simulink model "sliding_lin_working"  (R2015a)
settings: Solver=ode45  SolverMode=SingleTasking  StartTime=0.0  StopTime=Tsim
values from neighbouring files (symbols this model uses):
  EAd1 = 0    [Run_model.m]    (also in model_no_moments_getlinmod.m = EA_desired(1))
  EAd2 = 0    [Run_model.m]    (also in model_no_moments_getlinmod.m = EA_desired(2))
  EAd3 = 0    [Run_model.m]    (also in model_no_moments_getlinmod.m = EA_desired(3))
  EAinit1 = .5    (= 0.5)    [Run_model.m]
  EAinit2 = 1    [Run_model.m]
  EAinit3 = -1.3    [Run_model.m]
  Max_torque = thruster_torque + T_wheels    [Run_model.m]
  omd1 = 0    [Run_model.m]
  omd2 = 0    [Run_model.m]
  omd3 = 0    [Run_model.m]
  ominit1 = 2    [Run_model.m]
  ominit2 = 3    [Run_model.m]
  ominit3 = -4    [Run_model.m]
settings Model: CovMetricSettings=dwe  CovHtmlReporting=off  covSaveCumulativeToWorkspaceVar=off  CovSaveSingleToWorkspaceVar=off  CovExternalEMLEnable=on  Creator=hoddid  LastModifiedBy=hoddid
settings DataIOCC: LimitDataPoints=off  SaveFormat=Dataset
settings DebuggingCC: SFUnexpectedBacktrackingDiag=error  SFNoUnconditionalDefaultTransitionDiag=error
settings HardwareCC: ProdBitPerPointer=64  ProdLargestAtomicFloat=Float  ProdIntDivRoundTo=Zero  ProdEndianess=LittleEndian  ProdHWDeviceType=Specified
settings ModelReferenceCC: PropagateSignalLabelsOutOfModel=on
settings GRTTargetCC: TargetLangStandard=C99 (ISO)  GeneratePreprocessorConditionals=Use local settings

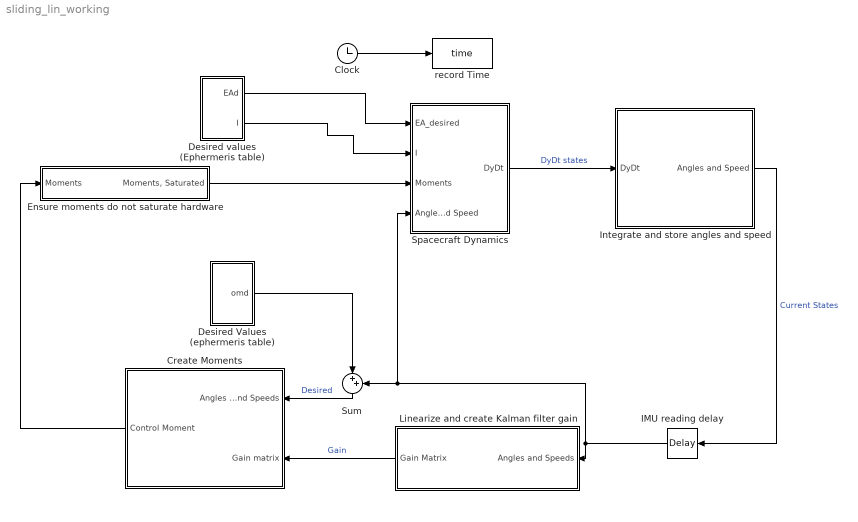
== system sliding_lin_working ==
  Clock : Clock
  Create Moments : Subsystem
  Desired Values (ephermeris table) : Subsystem
  Desired values (Ephermeris table) : Subsystem
  Ensure moments do not saturate hardware : Subsystem
  IMU reading delay : TransportDelay  DelayTime=0.0000001
  Integrate and store angles and speed : Subsystem
  Linearize and create Kalman filter gain : Subsystem
  Spacecraft Dynamics : Subsystem
  Sum : Sum  Inputs=|++
  record Time : ToWorkspace  VariableName=time  SampleTime=-1
      settings: Save2DSignal=2-D array (concatenate along first dimension)
  wires:
  Clock/1 -> record Time/1
  Integrate and store angles and speed/1(Angles and Speed) -> IMU reading delay/1  "Current States"
  Spacecraft Dynamics/1(DyDt) -> Integrate and store angles and speed/1(DyDt)  "DyDt states"
  Linearize and create Kalman filter gain/1(Gain Matrix) -> Create Moments/2(Gain matrix)  "Gain"
  Desired values (Ephermeris table)/1(EAd) -> Spacecraft Dynamics/1(EA_desired)
  Desired values (Ephermeris table)/2("I ") -> Spacecraft Dynamics/2(I)
  Create Moments/1(Control Moment) -> Ensure moments do not saturate hardware/1(Moments)
  Ensure moments do not saturate hardware/1("Moments, Saturated") -> Spacecraft Dynamics/3(Moments)
  Desired Values (ephermeris table)/1(omd) -> Sum/1
  Sum/1 -> Create Moments/1(Angles and Speeds)  "Desired"
  IMU reading delay/1 -> Sum/2, Spacecraft Dynamics/4(Angles and Speed), Linearize and create Kalman filter gain/1(Angles and Speeds)

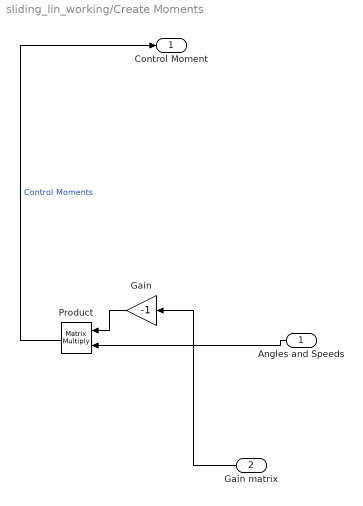
== system sliding_lin_working/Create Moments ==
  Angles and Speeds : Inport
  Gain matrix : Inport  Port=2
  Gain : Gain  Gain=-1
  Product : Product  Multiplication=Matrix(*)
  Control Moment : Outport
  wires:
  Angles and Speeds/1 -> Product/2
  Gain/1 -> Product/1
  Product/1 -> Control Moment/1  "Control Moments"
  Gain matrix/1 -> Gain/1

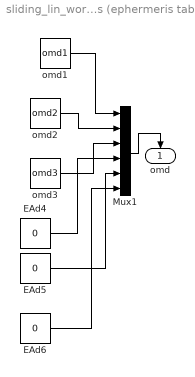
== system sliding_lin_working/Desired Values (ephermeris table) ==
  EAd4 : Constant  Value=0
  EAd5 : Constant  Value=0
  EAd6 : Constant  Value=0
  Mux1 : Mux  Inputs=6
  omd1 : Constant  Value=omd1
  omd2 : Constant  Value=omd2
  "omd3 " : Constant  Value=omd3
  omd : Outport
  wires:
  omd2/1 -> Mux1/2
  omd1/1 -> Mux1/1
  Mux1/1 -> omd/1
  "omd3 "/1 -> Mux1/3
  EAd5/1 -> Mux1/5
  EAd4/1 -> Mux1/4
  EAd6/1 -> Mux1/6

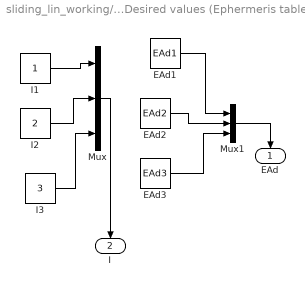
== system sliding_lin_working/Desired values (Ephermeris table) ==
  EAd1 : Constant  Value=EAd1
  EAd2 : Constant  Value=EAd2
  EAd3 : Constant  Value=EAd3
  I1 : Constant
  I2 : Constant  Value=2
  I3 : Constant  Value=3
  Mux : Mux  Inputs=3
  Mux1 : Mux  Inputs=3
  EAd : Outport
  "I " : Outport  Port=2
  wires:
  Mux/1 -> "I "/1
  EAd2/1 -> Mux1/2
  EAd1/1 -> Mux1/1
  I1/1 -> Mux/1
  Mux1/1 -> EAd/1
  I3/1 -> Mux/3
  I2/1 -> Mux/2
  EAd3/1 -> Mux1/3

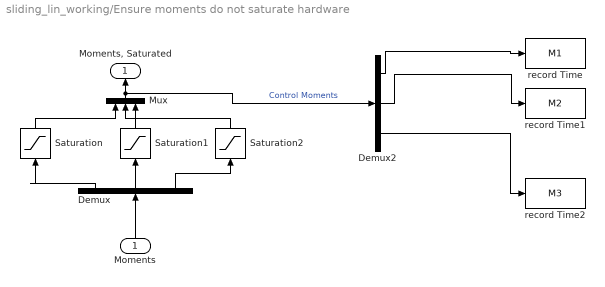
== system sliding_lin_working/Ensure moments do not saturate hardware ==
  Moments : Inport
  Demux : Demux  Outputs=3
  Demux2 : Demux  Outputs=3
  Mux : Mux  Inputs=3
  Saturation : Saturate  UpperLimit=Max_torque  LowerLimit=-Max_torque
  Saturation1 : Saturate  UpperLimit=Max_torque  LowerLimit=-Max_torque
  Saturation2 : Saturate  UpperLimit=Max_torque  LowerLimit=-Max_torque
  record Time : ToWorkspace  VariableName=M1  SampleTime=-1
      settings: Save2DSignal=2-D array (concatenate along first dimension)
  record Time1 : ToWorkspace  VariableName=M2  SampleTime=-1
      settings: Save2DSignal=2-D array (concatenate along first dimension)
  record Time2 : ToWorkspace  VariableName=M3  SampleTime=-1
      settings: Save2DSignal=2-D array (concatenate along first dimension)
  "Moments, Saturated" : Outport
  wires:
  Saturation1/1 -> Mux/2
  Demux/2 -> Saturation1/1
  Saturation2/1 -> Mux/3
  Demux/1 -> Saturation/1
  Saturation/1 -> Mux/1
  Demux/3 -> Saturation2/1
  Moments/1 -> Demux/1
  Mux/1 -> Demux2/1, "Moments, Saturated"/1  "Control Moments"
  Demux2/1 -> record Time/1
  Demux2/3 -> record Time2/1
  Demux2/2 -> record Time1/1

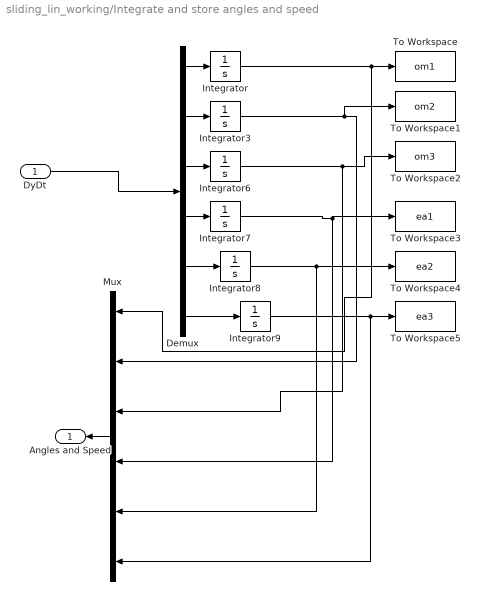
== system sliding_lin_working/Integrate and store angles and speed ==
  DyDt : Inport
  Demux : Demux  Outputs=6
  Integrator : Integrator  InitialCondition=ominit1
  Integrator3 : Integrator  InitialCondition=ominit2
  Integrator6 : Integrator  InitialCondition=ominit3
  Integrator7 : Integrator  InitialCondition=EAinit1
  Integrator8 : Integrator  InitialCondition=EAinit2
  Integrator9 : Integrator  InitialCondition=EAinit3
  Mux : Mux  Inputs=6
  To Workspace : ToWorkspace  VariableName=om1  SampleTime=-1
      settings: Save2DSignal=2-D array (concatenate along first dimension)
  To Workspace1 : ToWorkspace  VariableName=om2  SampleTime=-1
      settings: Save2DSignal=2-D array (concatenate along first dimension)
  To Workspace2 : ToWorkspace  VariableName=om3  SampleTime=-1
      settings: Save2DSignal=2-D array (concatenate along first dimension)
  To Workspace3 : ToWorkspace  VariableName=ea1  SampleTime=-1
      settings: Save2DSignal=2-D array (concatenate along first dimension)
  To Workspace4 : ToWorkspace  VariableName=ea2  SampleTime=-1
      settings: Save2DSignal=2-D array (concatenate along first dimension)
  To Workspace5 : ToWorkspace  VariableName=ea3  SampleTime=-1
      settings: Save2DSignal=2-D array (concatenate along first dimension)
  Angles and Speed : Outport
  wires:
  DyDt/1 -> Demux/1
  Demux/3 -> Integrator6/1
  Demux/1 -> Integrator/1
  Integrator7/1 -> Mux/4, To Workspace3/1
  Mux/1 -> Angles and Speed/1
  Integrator6/1 -> Mux/3, To Workspace2/1
  Integrator3/1 -> Mux/2, To Workspace1/1
  Demux/5 -> Integrator8/1
  Demux/6 -> Integrator9/1
  Demux/2 -> Integrator3/1
  Integrator8/1 -> Mux/5, To Workspace4/1
  Integrator9/1 -> Mux/6, To Workspace5/1
  Integrator/1 -> Mux/1, To Workspace/1
  Demux/4 -> Integrator7/1

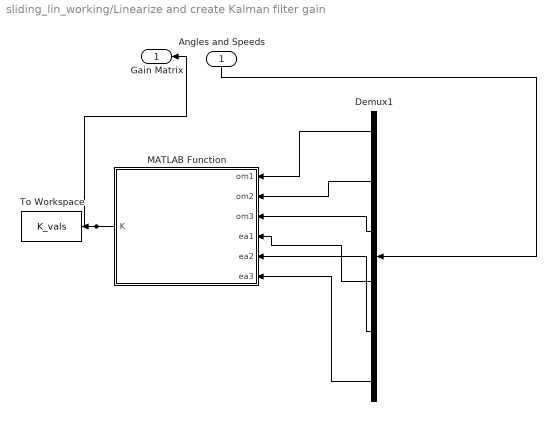
== system sliding_lin_working/Linearize and create Kalman filter gain ==
  Angles and Speeds : Inport
  Demux1 : Demux  Outputs=6
  MATLAB Function : MATLAB Function  TreatAsAtomicUnit=on
  To Workspace : ToWorkspace  VariableName=K_vals  SampleTime=-1
      settings: Save2DSignal=2-D array (concatenate along first dimension)
  Gain Matrix : Outport
  wires:
  Demux1/5 -> MATLAB Function/5(ea2)
  Demux1/3 -> MATLAB Function/3(om3)
  Demux1/1 -> MATLAB Function/1(om1)
  Demux1/2 -> MATLAB Function/2(om2)
  Demux1/4 -> MATLAB Function/4(ea1)
  Demux1/6 -> MATLAB Function/6(ea3)
  MATLAB Function/1(K) -> Gain Matrix/1, To Workspace/1
  Angles and Speeds/1 -> Demux1/1

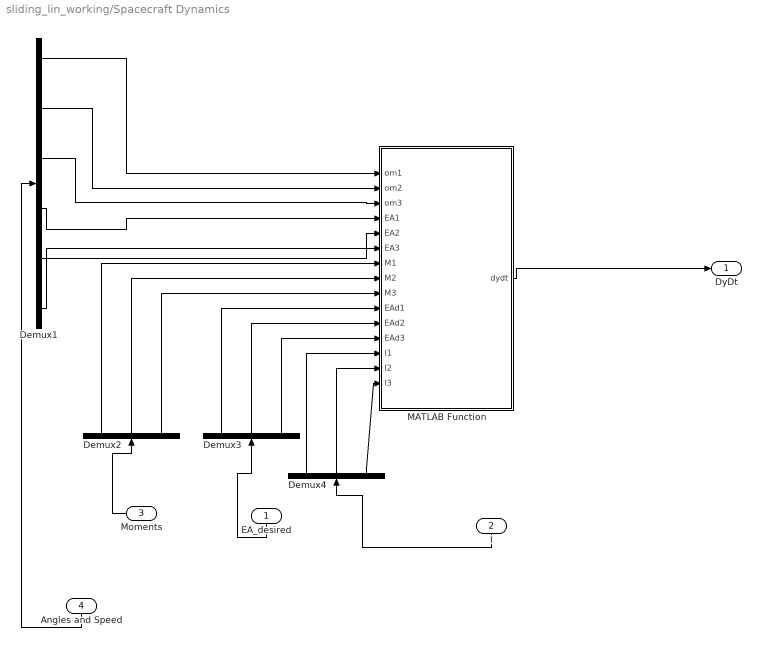
== system sliding_lin_working/Spacecraft Dynamics ==
  EA_desired : Inport
  I : Inport  Port=2
  Moments : Inport  Port=3
  Angles and Speed : Inport  Port=4
  Demux1 : Demux  Outputs=6
  Demux2 : Demux  Outputs=3
  Demux3 : Demux  Outputs=3
  Demux4 : Demux  Outputs=3
  MATLAB Function : MATLAB Function  TreatAsAtomicUnit=on
  DyDt : Outport
  wires:
  Demux2/1 -> MATLAB Function/7(M1)
  Demux2/3 -> MATLAB Function/9(M3)
  Demux2/2 -> MATLAB Function/8(M2)
  Demux1/5 -> MATLAB Function/5(EA2)
  Demux1/6 -> MATLAB Function/6(EA3)
  Demux1/1 -> MATLAB Function/1(om1)
  Demux1/2 -> MATLAB Function/2(om2)
  Demux1/4 -> MATLAB Function/4(EA1)
  Demux1/3 -> MATLAB Function/3(om3)
  Angles and Speed/1 -> Demux1/1
  MATLAB Function/1(dydt) -> DyDt/1
  Moments/1 -> Demux2/1
  Demux3/1 -> MATLAB Function/10(EAd1)
  Demux3/2 -> MATLAB Function/11(EAd2)
  Demux3/3 -> MATLAB Function/12(EAd3)
  EA_desired/1 -> Demux3/1
  Demux4/1 -> MATLAB Function/13(I1)
  Demux4/2 -> MATLAB Function/14(I2)
  Demux4/3 -> MATLAB Function/15(I3)
  I/1 -> Demux4/1

== matlab function sliding_lin_working/Linearize and create Kalman filter gain/MATLAB Function ==
  data: om1 input; K output; om2 input; om3 input; ea1 input; ea2 input; ea3 input
function K = linearize_get_Gain(om1,om2,om3,ea1,ea2,ea3)
%This Code takes in the current states, linearizes about them, 
% and returns the optimal gain matrix, K.

%create states:
om = [om1;om2;om3];
EA = [ea1; ea2; ea3];
Y0 = cat(1,om,EA);
T = [0;0;0]; % assume no moments

%get your A and B matricies via creating the Ax+b = Xdot state-space
%linearization
[A,B] = GetLinModFtxu_rolling(@model_no_moments_getlinmod,[],Y0,T);
C = eye(6);
D = zeros(6,3);
%these values must be tuned to acheive good control
R = 1;
Q1 = 1;
Q = 100*[Q1 0 0 0 0 0;
    0 Q1 0 0 0 0;
    0 0 Q1 0 0 0;
    0 0 0 Q1 0 0;
    0 0 0 0 Q1 0;
    0 0 0 0 0 Q1];
R = eye(3);

%declare the coder to be extrinsic so Simulink Can perform it
coder.extrinsic('lqr'); 
K = zeros(3,6);
%get Gain MAtrix
K = lqr(A,B,Q,R);
end

== matlab function sliding_lin_working/Spacecraft Dynamics/MATLAB Function ==
  data: om1 input; om2 input; om3 input; EA1 input; EA2 input; EA3 input; dydt output; M1 input; M2 input; M3 input; EAd1 input; EAd2 input; EAd3 input; I1 input; I2 input; I3 input
function dydt = fcn(om1,om2,om3,EA1,EA2,EA3,M1,M2,M3,EAd1,EAd2,EAd3,I1,I2,I3)
% Determine the derivative of the state

EA_desired = [EAd1;EAd2;EAd3;];
I = [I1;I2;I3;];

%% Update variables
om=[om1;om2;om3;];
EA = [EA1;EA2;EA3;];

%% Make Current SPACE123 DCM
EA1=EA(1);
EA2=EA(2);
EA3=EA(3);
C11=cos(EA2)*cos(EA3);
C12=cos(EA2)*sin(EA3);
C13=-sin(EA2);
C21=sin(EA1)*sin(EA2)*cos(EA3)-cos(EA1)*sin(EA3);
C22=sin(EA1)*sin(EA2)*sin(EA3)+cos(EA1)*cos(EA3);
C23=sin(EA1)*cos(EA2);
C31=cos(EA1)*sin(EA2)*cos(EA3)+sin(EA1)*sin(EA3);
C32=cos(EA1)*sin(EA2)*sin(EA3)-sin(EA1)*cos(EA3);
C33=cos(EA1)*cos(EA2);
DCM_actual=[C11 C12 C13; C21 C22 C23; C31 C32 C33];   
   

%% Make Desiried orientation-SPACE123 DCM
EAd1=EA_desired(1);
EAd2=EA_desired(2);
EAd3=EA_desired(3);
C11d=cos(EAd2)*cos(EAd3);
C12d=cos(EAd2)*sin(EAd3);
C13d=-sin(EAd2);
C21d=sin(EAd1)*sin(EAd2)*cos(EAd3)-cos(EAd1)*sin(EAd3);
C22d=sin(EAd1)*sin(EAd2)*sin(EAd3)+cos(EAd1)*cos(EAd3);
C23d=sin(EAd1)*cos(EAd2);
C31d=cos(EAd1)*sin(EAd2)*cos(EAd3)+sin(EAd1)*sin(EAd3);
C32d=cos(EAd1)*sin(EAd2)*sin(EAd3)-sin(EAd1)*cos(EAd3);
C33d=cos(EAd1)*cos(EAd2);
DCM_desired=[C11d C12d C13d; C21d C22d C23d; C31d C32d C33d];

%% Get Derivatives
% Spacecraft Euler's Equations
I1 = I(1);
I2 = I(2);
I3 = I(3);

om1=om(1);
om2=om(2);
om3=om(3);
omdot1=(M1+(I2-I3)*om2*om3)/I1;
omdot2=(M2+(I3-I1)*om3*om1)/I2;
omdot3=(M3+(I1-I2)*om1*om2)/I3;
omdot=[omdot1; omdot2; omdot3];

%% kinematic differential equations of motion
EA1=EA(1);
EA2=EA(2);
EA3=EA(3);

EAdot1=(1/cos(EA2))*(om1*cos(EA2)+om2*sin(EA1)*sin(EA2)+om3*cos(EA1)*sin(EA2));
EAdot2=(1/cos(EA2))*(om2*cos(EA1)*cos(EA2)-om3*sin(EA1)*cos(EA2));
EAdot3=(1/cos(EA2))*(om2*sin(EA1)+om3*cos(EA1));
EAdot=[EAdot1; EAdot2; EAdot3];

% specify state derivative values
dydt= cat(1,omdot,EAdot);
end
